simulink model "GalvoDiskPIDeinzel"  (R2013a)
settings: Solver=ode45  StartTime=0.0  StopTime=init.StopTime  MinStep=init.MinStepSize  RelTol=1e-3
model workspace: external: MAT-File /home/mainster/CODES_local/matlab_workspace/paramPID1.mat (data not in the file)
values from neighbouring files (symbols this model uses):
  init = struct('TsSens',   30e-6,              'TsSens2',  30e-6,              'StopTime', 50e-3,              'MinStepSize',  1e-6,              'DelayTime',    10e-6)    [GalvoTransferFuncFeedbackDelay_processing.m]    (also in GalvoTransferFuncFeedback_processing.m = struct('TsSens',   70e-6,              'TsSens2',  555e-6,  ; Galvo_process_analyze.m = 0)
  PID = sym2tf(eval(pid))    [GalvoModel_v4_sys.m]    (also in GalvoModel_v6_sys.m; GalvoTransferFuncFeedbackDelay_processing.m = struct( 'P',    0.392064644185526,              'I',    2068)
undefined symbols (not defined in the file or in its folder): DiscIntNeverNeededParam
libraries: simulink x2
settings Model: Creator=mainster  LastModifiedBy=mainster

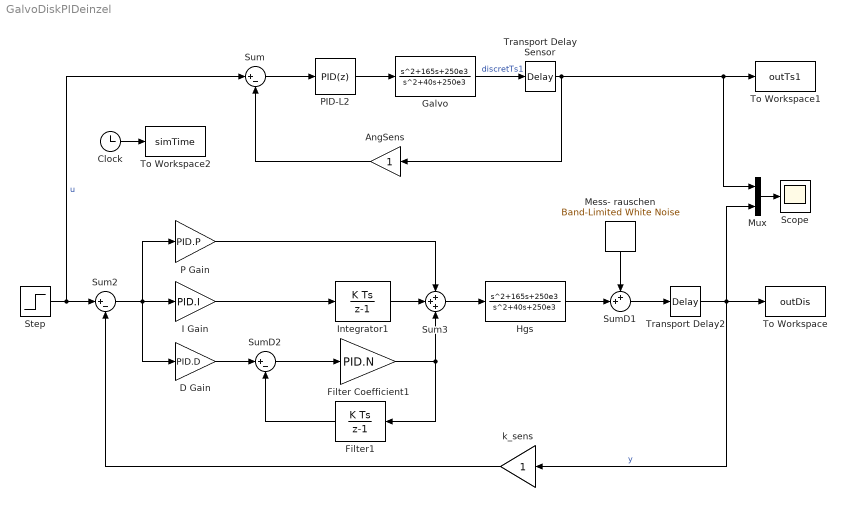
== system GalvoDiskPIDeinzel ==
  AngSens : Gain  SampleTime=init.TsSens
  Clock : Clock
  "D Gain " : Gain  DisableCoverage=on  Gain=PID.D  OutDataTypeStr=Inherit: Inherit via back propagation  SampleTime=PID.Ts
  Filter Coefficient1 : Gain  Gain=PID.N  OutDataTypeStr=Inherit: Inherit via back propagation  SampleTime=PID.Ts
  Filter1 : DiscreteIntegrator  DisableCoverage=on  InitialConditionMode=State only (most efficient)  SampleTime=PID.Ts  OutDataTypeStr=Inherit: Inherit via back propagation  ICPrevOutput=DiscIntNeverNeededParam  ICPrevScaledInput=DiscIntNeverNeededParam
  Galvo : TransferFcn  Numerator=[1 165 250e3]  Denominator=[1 40 250e3]
  Hgs : TransferFcn  Numerator=[1 165 250e3]  Denominator=[1 40 250e3]
  "I Gain " : Gain  DisableCoverage=on  Gain=PID.I  OutDataTypeStr=Inherit: Inherit via back propagation  SampleTime=PID.Ts
  Integrator1 : DiscreteIntegrator  InitialConditionMode=State only (most efficient)  SampleTime=PID.Ts  OutDataTypeStr=Inherit: Inherit via back propagation  ICPrevOutput=DiscIntNeverNeededParam  ICPrevScaledInput=DiscIntNeverNeededParam
  Mess- rauschen : simulink/Sources/Band-Limited White Noise  Cov=[0.1e-15]  Ts=0  seed=[23341]
  Mux : Mux  Inputs=2
  P Gain : Gain  Gain=PID.P  SampleTime=PID.Ts
  PID-L2 : simulink/Continuous/PID Controller  Controller=PID  TimeDomain=Discrete-time  SampleTime=PID.Ts  IntegratorMethod=Forward Euler  FilterMethod=Forward Euler  Form=Parallel  P=0.384349742528594  I=2468.66636470386  D=0  N=100  InitialConditionSource=internal  InitialConditionForIntegrator=0  InitialConditionForFilter=0  ExternalReset=none  LimitOutput=off  UpperSaturationLimit=inf  LowerSaturationLimit=-inf  LinearizeAsGain=off  AntiWindupMode=none  Kb=1  TrackingMode=off  Kt=1  PParamMin=[]  PParamMax=[]  IParamMin=[]  IParamMax=[]  DParamMin=[]  DParamMax=[]  NParamMin=[]  NParamMax=[]  KbParamMin=[]  KbParamMax=[]  KtParamMin=[]  KtParamMax=[]  POutMin=[]  POutMax=[]  IOutMin=[]  IOutMax=[]  DOutMin=[]  DOutMax=[]  NOutMin=[]  NOutMax=[]  KbOutMin=[]  KbOutMax=[]  KtOutMin=[]  KtOutMax=[]  IntegratorOutMin=[]  IntegratorOutMax=[]  FilterOutMin=[]  FilterOutMax=[]  SumOutMin=[]  SumOutMax=[]  SumI1OutMin=[]  SumI1OutMax=[]  SumI2OutMin=[]  SumI2OutMax=[]  SumI3OutMin=[]  SumI3OutMax=[]  SumDOutMin=[]  SumDOutMax=[]  SaturationOutMin=[]  SaturationOutMax=[]  IntegratorContinuousStateAttributes=''  IntegratorStateMustResolveToSignalObject=off  IntegratorRTWStateStorageClass=Auto  FilterContinuousStateAttributes=''  FilterStateMustResolveToSignalObject=off  FilterRTWStateStorageClass=Auto
  Scope : Scope
  Step : Step  Time=5e-3  SampleTime=0
  Sum : Sum  Inputs=|+-  SampleTime=init.TsSens
  Sum2 : Sum  Inputs=|+-  SampleTime=init.TsSens
  Sum3 : Sum  Inputs=+++  OutDataTypeStr=Inherit: Inherit via back propagation  SampleTime=PID.Ts
  SumD1 : Sum  DisableCoverage=on  Inputs=++|
  SumD2 : Sum  DisableCoverage=on  Inputs=|+-  SampleTime=PID.Ts
  To Workspace : ToWorkspace  VariableName=outDis  SampleTime=-1  SaveFormat=Timeseries
  To Workspace1 : ToWorkspace  VariableName=outTs1  SampleTime=-1  SaveFormat=Timeseries
  To Workspace2 : ToWorkspace  VariableName=simTime  SampleTime=-1  SaveFormat=Timeseries
  Transport Delay Sensor : TransportDelay  DelayTime=init.DelayTime
  Transport Delay2 : TransportDelay  DelayTime=init.DelayTime
  k_sens : Gain  SampleTime=init.TsSens
  wires:
  Sum/1 -> PID-L2/1
  Galvo/1 -> Transport Delay Sensor/1  "discretTs1"
  PID-L2/1 -> Galvo/1
  AngSens/1 -> Sum/2
  Transport Delay Sensor/1 -> AngSens/1, Mux/1, To Workspace1/1
  Transport Delay2/1 -> Mux/2, To Workspace/1, k_sens/1  "y"
  k_sens/1 -> Sum2/2
  Hgs/1 -> SumD1/2
  SumD1/1 -> Transport Delay2/1
  Mess- rauschen/1 -> SumD1/1
  Step/1 -> Sum/1, Sum2/1  "u"
  "I Gain "/1 -> Integrator1/1
  "D Gain "/1 -> SumD2/1
  SumD2/1 -> Filter Coefficient1/1
  Filter Coefficient1/1 -> Sum3/3, Filter1/1
  Filter1/1 -> SumD2/2
  Integrator1/1 -> Sum3/2
  P Gain/1 -> Sum3/1
  Sum3/1 -> Hgs/1
  Sum2/1 -> P Gain/1, "I Gain "/1, "D Gain "/1
  Mux/1 -> Scope/1
  Clock/1 -> To Workspace2/1
